simulink model "comp_mdl"  (R2021b)
settings: Solver=ode1  StartTime=0.0  StopTime=10  FixedStep=0.001  MaxStep=0.1  MinStep=0.001  RelTol=1e-3  EnableMultiTasking=on
values from neighbouring files (symbols this model uses):
  A = [0 1; 0 0]    [pendulum_data.m]
  B = [0;1]    [pendulum_data.m]
  C = C([1,3],:)    [comp_data.m]    (also in pendulum_data.m = [1 1])
  delta = 0.001    [comp_data.m]    (also in obsint_data.m; obsmod_data.m; outmod_data.m; outmodc_data.m)
  L = -inv(S*B)*(S*Am-Phi*S)    [stmod_data.m]
  rho = 1    [comp_data.m]    (also in obsint_data.m; obsmod_data.m; outmod_data.m; outmodc_data.m)
  S = rpp(A,B,psm)    [obsint_data.m]    (also in stint_data.m = rpp(A,B,sp); stmod_data.m = inv(S*B)*S; streg_data.m = rpp(A,B,sp))
  x0 = zeros(1,n)    [comp_data.m]    (also in obsint_data.m; obsmod_data.m; outmod_data.m; outmodc_data.m)
  xc0 = zeros(1,n-p)    [comp_data.m]    (also in obsmod_data.m; outmodc_data.m)
undefined symbols (not defined in the file or in its folder): Dhat, Hhat, Lam, m, n, p, P
settings Model: Creator=w.schwamm  LastModifiedBy=Witali
settings SolverCC: AlgebraicLoopSolver=TrustRegion
settings DataIOCC: SaveOutput=off  SaveTime=off  ReturnWorkspaceOutputs=off  StateSaveName=x  TimeSaveName=t  OutputSaveName=y
settings OptimizationCC: LifeSpan=inf
settings DebuggingCC: SFUnexpectedBacktrackingDiag=warning  SFNoUnconditionalDefaultTransitionDiag=warning  SFMachineParentedDataDiag=warning  ArithmeticOperatorsInVariantConditions=warning
settings SFSimCC: SimUseLocalCustomCode=off  CustomCodeUndefinedFunction=UseInterfaceOnly
settings RTWCC: RTWUseLocalCustomCode=off
settings CodeAppCC: StateflowObjectComments=on
settings GRTTargetCC: TargetLangStandard=C89/C90 (ANSI)
settings ConfigComp: CovMetricSettings=dw  CovSaveCumulativeToWorkspaceVar=on  CovSaveSingleToWorkspaceVar=on  CovExternalEMLEnable=off

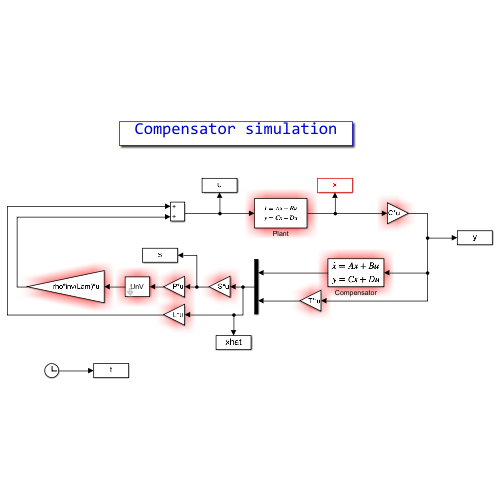
[thumbnail: Simulink's stored preview of the top-level diagram]
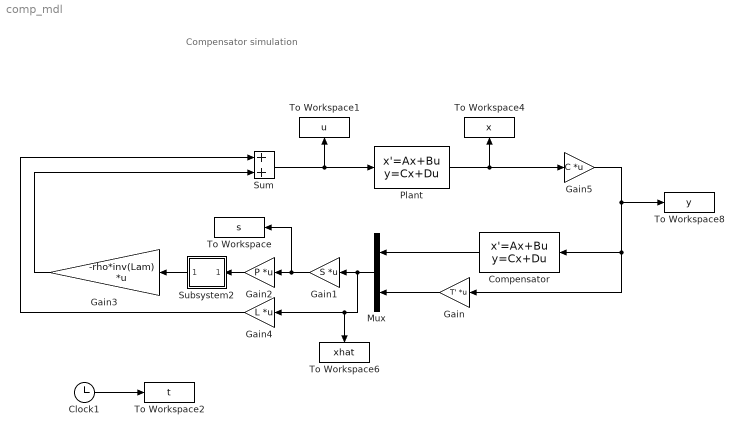
== system comp_mdl ==
  note: Compensator simulation
  Clock1 : Clock
  Compensator : StateSpace  A=Hhat  B=Dhat  C=eye(n-p)  D=zeros(n-p,p)  InitialCondition=xc0
  Gain : Gain  Gain=T'  Multiplication=Matrix(K*u)
  Gain1 : Gain  Gain=S  Multiplication=Matrix(K*u)
  Gain2 : Gain  Gain=P  Multiplication=Matrix(K*u)
  Gain3 : Gain  Gain=-rho*inv(Lam)  Multiplication=Matrix(K*u)
  Gain4 : Gain  Gain=L  Multiplication=Matrix(K*u)
  Gain5 : Gain  Gain=C  Multiplication=Matrix(K*u)
  Mux : Mux  Inputs=2
  Plant : StateSpace  A=A  B=B  C=eye(n)  D=zeros(n,m)  InitialCondition=x0
  Subsystem2 : Subsystem  mask{delta=delta}
      mask prompts: delta "Unit vector delta:"
      mask Display: disp('UnV')
  Sum : Sum  InputSameDT=on  SaturateOnIntegerOverflow=on  OutDataTypeStr=Inherit: Same as first input
  To Workspace : ToWorkspace  VariableName=s  SaveFormat=Timeseries  SampleTime=-1
      settings: MaxDataPoints=1000000
  To Workspace1 : ToWorkspace  VariableName=u  SaveFormat=Timeseries  SampleTime=-1
      settings: MaxDataPoints=1000000
  To Workspace2 : ToWorkspace  VariableName=t  SaveFormat=Timeseries  SampleTime=-1
      settings: MaxDataPoints=1000000
  To Workspace4 : ToWorkspace  VariableName=x  SaveFormat=Timeseries  SampleTime=-1
      settings: MaxDataPoints=1000000
  To Workspace6 : ToWorkspace  VariableName=xhat  SaveFormat=Timeseries  SampleTime=-1
      settings: MaxDataPoints=1000000
  To Workspace8 : ToWorkspace  VariableName=y  SaveFormat=Timeseries  SampleTime=-1
      settings: MaxDataPoints=1000000
  wires:
  Plant/1 -> Gain5/1, To Workspace4/1
  Clock1/1 -> To Workspace2/1
  Gain5/1 -> Compensator/1, Gain/1, To Workspace8/1
  Subsystem2/1(Out1) -> Gain3/1
  Mux/1 -> To Workspace6/1, Gain4/1, Gain1/1
  Gain/1 -> Mux/2
  Compensator/1 -> Mux/1
  Gain1/1 -> Gain2/1, To Workspace/1
  Gain2/1 -> Subsystem2/1(In1)
  Gain4/1 -> Sum/1
  Gain3/1 -> Sum/2
  Sum/1 -> Plant/1, To Workspace1/1

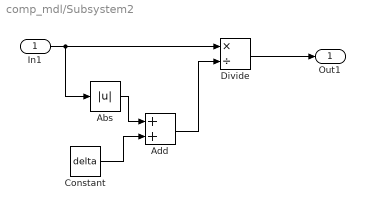
== system comp_mdl/Subsystem2 ==
  In1 : Inport
  Abs : Abs
  Add : Sum
  Constant : Constant  Value=delta  SampleTime=-1
  Divide : Product  Inputs=*/
  Out1 : Outport
  wires:
  Constant/1 -> Add/2
  Add/1 -> Divide/2
  Abs/1 -> Add/1
  Divide/1 -> Out1/1
  In1/1 -> Divide/1, Abs/1
